simulink model "model"  (R2025b)
settings: Solver=VariableStepAuto  StartTime=0.0  StopTime=10.0  RelTol=1e-3
undefined symbols (not defined in the file): G_den, G_num
settings Model: Creator=nuris  LastModifiedBy=nuris

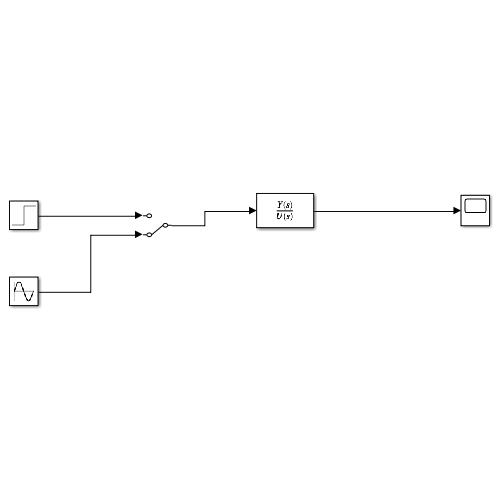
[thumbnail: Simulink's stored preview of the top-level diagram]
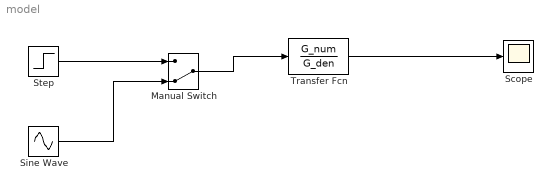
== system model ==
  Manual Switch : ManualSwitch  CurrentSetting=0
  Scope : Scope
      settings: ActiveDisplayYMinimum=-1.0275047937889008  ActiveDisplayYMaximum=1.0266993255516763
  Sine Wave : Sin  Amplitude=5  Frequency=2  SampleTime=0
  Step : Step  SampleTime=0
  Transfer Fcn : TransferFcn  Numerator=G_num  Denominator=G_den
  wires:
  Transfer Fcn/1 -> Scope/1
  Step/1 -> Manual Switch/1
  Manual Switch/1 -> Transfer Fcn/1
  Sine Wave/1 -> Manual Switch/2
